simulink model "unicycle_kin_trajCont_test_1"  (R2020a)
settings: Solver=FixedStepAuto  StartTime=0.0  StopTime=inf  RelTol=1e-3
undefined symbols (not defined in the file): X, Y
libraries: robotlib x5

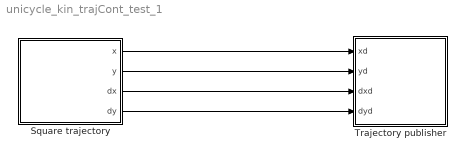
== system unicycle_kin_trajCont_test_1 ==
  Square trajectory : Subsystem  mask{L=3, v=0.2, start=[0,0]}
      mask prompts: L "Side length"; v "Speed"; start "Start position [x, y]"
  Trajectory publisher : Subsystem  mask{simPublishRate=10}
      mask prompts: simPublishRate "Publising rate [Hz]"
  wires:
  Square trajectory/1(x) -> Trajectory publisher/1(xd)
  Square trajectory/2(y) -> Trajectory publisher/2(yd)
  Square trajectory/3(dx) -> Trajectory publisher/3(dxd)
  Square trajectory/4(dy) -> Trajectory publisher/4(dyd)

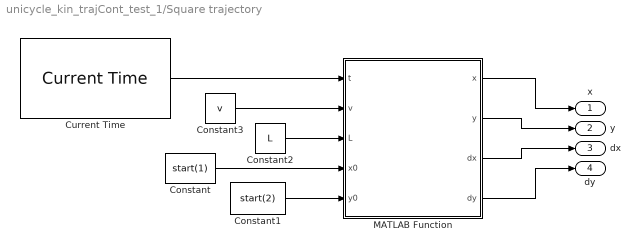
== system unicycle_kin_trajCont_test_1/Square trajectory ==
  Constant : Constant  Value=start(1)
  Constant1 : Constant  Value=start(2)
  Constant2 : Constant  Value=L
  Constant3 : Constant  Value=v
  Current Time : robotlib/Current Time  OutputFormat=double  SampleTime=-1  ModelName=unicycle_kin_trajCont_test_1
  MATLAB Function : MATLAB Function  TreatAsAtomicUnit=on
  x : Outport
  y : Outport  Port=2
  dx : Outport  Port=3
  dy : Outport  Port=4
  wires:
  MATLAB Function/2(y) -> y/1
  Constant3/1 -> MATLAB Function/2(v)
  Constant2/1 -> MATLAB Function/3(L)
  Constant1/1 -> MATLAB Function/5(y0)
  MATLAB Function/3(dx) -> dx/1
  MATLAB Function/4(dy) -> dy/1
  Current Time/1 -> MATLAB Function/1(t)
  Constant/1 -> MATLAB Function/4(x0)
  MATLAB Function/1(x) -> x/1

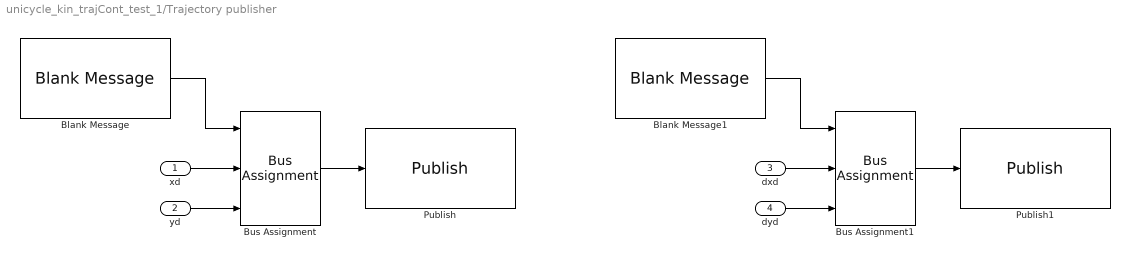
== system unicycle_kin_trajCont_test_1/Trajectory publisher ==
  xd : Inport  SampleTime=1/simPublishRate
  yd : Inport  Port=2  SampleTime=1/simPublishRate
  dxd : Inport  Port=3  SampleTime=1/simPublishRate
  dyd : Inport  Port=4  SampleTime=1/simPublishRate
  Blank Message : robotlib/Blank Message  messageClass=Message  entityType=geometry_msgs/Point  messageType=geometry_msgs/Point  SampleTime=1/simPublishRate
  Blank Message1 : robotlib/Blank Message  messageClass=Message  entityType=geometry_msgs/Point  messageType=geometry_msgs/Point  SampleTime=1/simPublishRate
  Bus Assignment : BusAssignment  AssignedSignals=X,Y
  Bus Assignment1 : BusAssignment  AssignedSignals=X,Y
  Publish : robotlib/Publish  topicSource=Specify your own  topic=/desired_position  messageType=geometry_msgs/Point  messageQueueLength=1
  Publish1 : robotlib/Publish  topicSource=Specify your own  topic=/desired_velocity  messageType=geometry_msgs/Point  messageQueueLength=1
  wires:
  Bus Assignment/1 -> Publish/1
  Blank Message/1 -> Bus Assignment/1
  xd/1 -> Bus Assignment/2
  yd/1 -> Bus Assignment/3
  dyd/1 -> Bus Assignment1/3
  dxd/1 -> Bus Assignment1/2
  Blank Message1/1 -> Bus Assignment1/1
  Bus Assignment1/1 -> Publish1/1

== matlab function unicycle_kin_trajCont_test_1/Square trajectory/MATLAB Function ==
function [x,y,dx,dy] = square_trajectory(t,v,L,x0,y0)

if (t<L/v)
    x = x0+v*t;
    y = y0;
    dx = v;
    dy = 0;
elseif (t>=L/v) && (t<2*L/v)
    x = x0+L;
    y = y0+v*(t-L/v);
    dx = 0;
    dy = v;
elseif (t>=2*L/v) && (t<3*L/v)
    x = x0+L-v*(t-2*L/v);
    y = y0+L;
    dx = -v;
    dy = 0;
elseif (t>=3*L/v) && (t<4*L/v)
    x = x0;
    y = y0+L-v*(t-3*L/v);
    dx = 0;
    dy = -v;
else
    x = x0;
    y = y0;
    dx = 0;
    dy = 0;
end
